simulink model "BLDCmotorControl_FOC_R2017b_fixdt_Ffwd"  (R2025a)
settings: Solver=FixedStepDiscrete  StartTime=0  StopTime=0.5  FixedStep=Ts  MaxStep=1e-6  RelTol=1e-6  AbsTol=1e-6  EnableMultiTasking=on
PreLoadFcn:
  | addpath(genpath('01_Libraries'));
  | addpath(genpath('02_Figures'));
InitFcn:
  | init_model;
undefined symbols (not defined in the file): a_elecAngle, b_DCLinkCurrAvail, b_diagEna, b_FfwdEna, b_fieldWeakEna, b_selPhaABCurrMeas, cf_currFilt, cf_speedCoef, cf_speedFilt, CTRL_COM, DiscIntNeverNeededParam, dV_openRate, DWORK0, DWORK1, DWORK2, DWORK3, dz_cntTrnsDetHi, dz_cntTrnsDetLo, i_errThres, i_max, i_thresOutlier, id_fieldWeak_M1, id_Kb, id_Ki, id_Kp, iq_Kb, iq_Ki, iq_KiLimProt, iq_Kp, iq_KpLimProt, iq_max_M1, Ld, Lq, mot_lambda, mot_Ld, mot_Lq, n_commAcvLo, n_commDeacvHi, n_Kb, n_Ki, n_Kp, n_KpLimProt, n_max, n_stdStillDet, OPEN_MODE, r_cos_M1, r_sin_M1, r_whl, Rs, SPD_MODE, t_errDequal, t_errQual, TRQ_MODE, Ts, Ts_ctrl, V_max, V_min, Vd_max, vec_hallToPos, VLT_MODE ... (+5)
libraries: BLDC_controller_Lib x12, simulink x11, spsPermanentMagnetSynchronousMachineLib x4, spsVoltageMeasurementLib x4, spsControlledVoltageSourceLib x2, spsUniversalBridgeLib x2, spspowerguiLib x2, eePwmGenerator x1, SignalEditorBlockLib x1
(part 2 of 4)

== system BLDCmotorControl_FOC_R2017b_fixdt_Ffwd/PWM_gates/PWM_generator12 ==
  DC : Inport  SampleTime=Ts
  PWM_generator_sfcn : S-Function  FunctionName=PWM_generator_sf  SFunctionModules=""  SFunctionDeploymentMode=off  EnableBusSupport=off  SFcnStateName=DWORK0  mask{rtw_sf_name=PWM_generator_sf, showVar=off}
      mask prompts: rtw_sf_name "Simulink:masks:GenSFuncName_MP"; showVar "Simulink:masks:GenSFuncShowModuleList_MP"
      mask help: Simulink:masks:GenSFuncDesc_MD
      mask init: same as BLDCmotorControl_FOC_R2017b_fixdt_Ffwd/BLDC_model_closed/BLDC_model_sfcn
      settings: SFcnIsStateOwnerBlock=on
      settings: CopyFcn=|
      | if ~strcmp(get_param(gcb,'Linkstatus'),'none') && ...
      | ~strcmp(get_param(gcb,'Linkstatus'),'implicit')
      |   set_param(gcb,'LinkStatus','none');
      | end
      mask Help: eval('feval(''rtwprivate'',''rtwhelpview'',''rtw_sfcn_block'')');
      mask Display:
      | port_label('input',1,'DC');
      | port_label('output',1,'PWM');
  __InputSSForSFun__ : Subsystem
  __OutputSSForSFun__ : Subsystem
  PWM : Outport  VectorParamsAs1DForOutWhenUnconnected=off
  wires:
  DC/1 -> __InputSSForSFun__/1(DC)
  __InputSSForSFun__/1(__UniqueOutportName__1__) -> PWM_generator_sfcn/1
  PWM_generator_sfcn/1 -> __OutputSSForSFun__/1(__UniqueInportName__1__)
  __OutputSSForSFun__/1(PWM) -> PWM/1

== system BLDCmotorControl_FOC_R2017b_fixdt_Ffwd/PWM_gates/PWM_generator2 ==
  DC : Inport  SampleTime=Ts
  PWM_generator_sfcn : S-Function  FunctionName=PWM_generator_sf  SFunctionModules=""  SFunctionDeploymentMode=off  EnableBusSupport=off  SFcnStateName=DWORK0  mask{rtw_sf_name=PWM_generator_sf, showVar=off}
      mask prompts: rtw_sf_name "Simulink:masks:GenSFuncName_MP"; showVar "Simulink:masks:GenSFuncShowModuleList_MP"
      mask help: Simulink:masks:GenSFuncDesc_MD
      mask init: same as BLDCmotorControl_FOC_R2017b_fixdt_Ffwd/BLDC_model_closed/BLDC_model_sfcn
      settings: SFcnIsStateOwnerBlock=on
      settings: CopyFcn=|
      | if ~strcmp(get_param(gcb,'Linkstatus'),'none') && ...
      | ~strcmp(get_param(gcb,'Linkstatus'),'implicit')
      |   set_param(gcb,'LinkStatus','none');
      | end
      mask Help: eval('feval(''rtwprivate'',''rtwhelpview'',''rtw_sfcn_block'')');
      mask Display:
      | port_label('input',1,'DC');
      | port_label('output',1,'PWM');
  __InputSSForSFun__ : Subsystem
  __OutputSSForSFun__ : Subsystem
  PWM : Outport  VectorParamsAs1DForOutWhenUnconnected=off
  wires:
  DC/1 -> __InputSSForSFun__/1(DC)
  __InputSSForSFun__/1(__UniqueOutportName__1__) -> PWM_generator_sfcn/1
  PWM_generator_sfcn/1 -> __OutputSSForSFun__/1(__UniqueInportName__1__)
  __OutputSSForSFun__/1(PWM) -> PWM/1

== system BLDCmotorControl_FOC_R2017b_fixdt_Ffwd/PWM_gates/PWM_generator3 ==
  DC : Inport  SampleTime=Ts
  PWM_generator_sfcn : S-Function  FunctionName=PWM_generator_sf  SFunctionModules=""  SFunctionDeploymentMode=off  EnableBusSupport=off  SFcnStateName=DWORK0  mask{rtw_sf_name=PWM_generator_sf, showVar=off}
      mask prompts: rtw_sf_name "Simulink:masks:GenSFuncName_MP"; showVar "Simulink:masks:GenSFuncShowModuleList_MP"
      mask help: Simulink:masks:GenSFuncDesc_MD
      mask init: same as BLDCmotorControl_FOC_R2017b_fixdt_Ffwd/BLDC_model_closed/BLDC_model_sfcn
      settings: SFcnIsStateOwnerBlock=on
      settings: CopyFcn=|
      | if ~strcmp(get_param(gcb,'Linkstatus'),'none') && ...
      | ~strcmp(get_param(gcb,'Linkstatus'),'implicit')
      |   set_param(gcb,'LinkStatus','none');
      | end
      mask Help: eval('feval(''rtwprivate'',''rtwhelpview'',''rtw_sfcn_block'')');
      mask Display:
      | port_label('input',1,'DC');
      | port_label('output',1,'PWM');
  __InputSSForSFun__ : Subsystem
  __OutputSSForSFun__ : Subsystem
  PWM : Outport  VectorParamsAs1DForOutWhenUnconnected=off
  wires:
  __OutputSSForSFun__/1(PWM) -> PWM/1
  PWM_generator_sfcn/1 -> __OutputSSForSFun__/1(__UniqueInportName__1__)
  __InputSSForSFun__/1(__UniqueOutportName__1__) -> PWM_generator_sfcn/1
  DC/1 -> __InputSSForSFun__/1(DC)

== system BLDCmotorControl_FOC_R2017b_fixdt_Ffwd/PWM_gates/PWM_generator4 ==
  DC : Inport  SampleTime=Ts
  PWM_generator_sfcn : S-Function  FunctionName=PWM_generator_sf  SFunctionModules=""  SFunctionDeploymentMode=off  EnableBusSupport=off  SFcnStateName=DWORK0  mask{rtw_sf_name=PWM_generator_sf, showVar=off}
      mask prompts: rtw_sf_name "Simulink:masks:GenSFuncName_MP"; showVar "Simulink:masks:GenSFuncShowModuleList_MP"
      mask help: Simulink:masks:GenSFuncDesc_MD
      mask init: same as BLDCmotorControl_FOC_R2017b_fixdt_Ffwd/BLDC_model_closed/BLDC_model_sfcn
      settings: SFcnIsStateOwnerBlock=on
      settings: CopyFcn=|
      | if ~strcmp(get_param(gcb,'Linkstatus'),'none') && ...
      | ~strcmp(get_param(gcb,'Linkstatus'),'implicit')
      |   set_param(gcb,'LinkStatus','none');
      | end
      mask Help: eval('feval(''rtwprivate'',''rtwhelpview'',''rtw_sfcn_block'')');
      mask Display:
      | port_label('input',1,'DC');
      | port_label('output',1,'PWM');
  __InputSSForSFun__ : Subsystem
  __OutputSSForSFun__ : Subsystem
  PWM : Outport  VectorParamsAs1DForOutWhenUnconnected=off
  wires:
  DC/1 -> __InputSSForSFun__/1(DC)
  __InputSSForSFun__/1(__UniqueOutportName__1__) -> PWM_generator_sfcn/1
  PWM_generator_sfcn/1 -> __OutputSSForSFun__/1(__UniqueInportName__1__)
  __OutputSSForSFun__/1(PWM) -> PWM/1

== system BLDCmotorControl_FOC_R2017b_fixdt_Ffwd/PWM_gates/PWM_generator5 ==
  DC : Inport  SampleTime=Ts
  PWM_generator_sfcn : S-Function  FunctionName=PWM_generator_sf  SFunctionModules=""  SFunctionDeploymentMode=off  EnableBusSupport=off  SFcnStateName=DWORK0  mask{rtw_sf_name=PWM_generator_sf, showVar=off}
      mask prompts: rtw_sf_name "Simulink:masks:GenSFuncName_MP"; showVar "Simulink:masks:GenSFuncShowModuleList_MP"
      mask help: Simulink:masks:GenSFuncDesc_MD
      mask init: same as BLDCmotorControl_FOC_R2017b_fixdt_Ffwd/BLDC_model_closed/BLDC_model_sfcn
      settings: SFcnIsStateOwnerBlock=on
      settings: CopyFcn=|
      | if ~strcmp(get_param(gcb,'Linkstatus'),'none') && ...
      | ~strcmp(get_param(gcb,'Linkstatus'),'implicit')
      |   set_param(gcb,'LinkStatus','none');
      | end
      mask Help: eval('feval(''rtwprivate'',''rtwhelpview'',''rtw_sfcn_block'')');
      mask Display:
      | port_label('input',1,'DC');
      | port_label('output',1,'PWM');
  __InputSSForSFun__ : Subsystem
  __OutputSSForSFun__ : Subsystem
  PWM : Outport  VectorParamsAs1DForOutWhenUnconnected=off
  wires:
  __OutputSSForSFun__/1(PWM) -> PWM/1
  PWM_generator_sfcn/1 -> __OutputSSForSFun__/1(__UniqueInportName__1__)
  __InputSSForSFun__/1(__UniqueOutportName__1__) -> PWM_generator_sfcn/1
  DC/1 -> __InputSSForSFun__/1(DC)

== system BLDCmotorControl_FOC_R2017b_fixdt_Ffwd/PWM_gates/signal_log6 ==
  PWM : Inport
  Terminator_1 : Terminator
  wires:
  PWM/1 -> Terminator_1/1  "PWM"

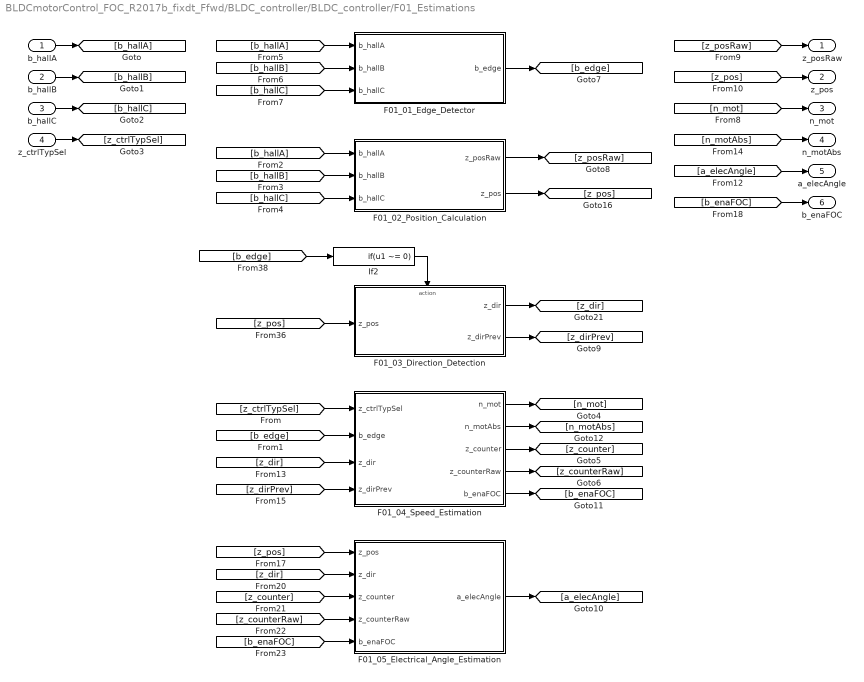
== system BLDCmotorControl_FOC_R2017b_fixdt_Ffwd/BLDC_controller/BLDC_controller/F01_Estimations ==
  b_hallA : Inport
  b_hallB : Inport  Port=2
  b_hallC : Inport  Port=3
  z_ctrlTypSel : Inport  Port=4
  F01_01_Edge_Detector : Subsystem
  F01_02_Position_Calculation : Subsystem
  F01_03_Direction_Detection : Subsystem
  F01_04_Speed_Estimation : Subsystem
  F01_05_Electrical_Angle_Estimation : Subsystem
  If2 : If  IfExpression=u1 ~= 0  ShowElse=off
  z_posRaw : Outport  OutputWhenDisabled=reset  InitialOutput=0  VectorParamsAs1DForOutWhenUnconnected=off
  z_pos : Outport  Port=2  OutputWhenDisabled=reset  InitialOutput=0  VectorParamsAs1DForOutWhenUnconnected=off
  "n_mot " : Outport  Port=3  OutputWhenDisabled=reset  InitialOutput=0  VectorParamsAs1DForOutWhenUnconnected=off
  n_motAbs : Outport  Port=4  OutputWhenDisabled=reset  InitialOutput=0  VectorParamsAs1DForOutWhenUnconnected=off
  a_elecAngle : Outport  Port=5  OutputWhenDisabled=reset  InitialOutput=0  VectorParamsAs1DForOutWhenUnconnected=off
  b_enaFOC : Outport  Port=6  VectorParamsAs1DForOutWhenUnconnected=off
  wires:
  If2/1 -> F01_03_Direction_Detection/Action
  [b_edge] -> If2/1
  [z_pos] -> F01_03_Direction_Detection/1(z_pos)
  [b_hallA] -> F01_01_Edge_Detector/1(b_hallA)
  F01_01_Edge_Detector/1("b_edge ") -> [b_edge]
  F01_03_Direction_Detection/1(z_dir) -> [z_dir]
  [b_hallB] -> F01_01_Edge_Detector/2(b_hallB)
  [b_hallC] -> F01_01_Edge_Detector/3(b_hallC)
  b_hallA/1 -> [b_hallA]
  b_hallB/1 -> [b_hallB]
  b_hallC/1 -> [b_hallC]
  [b_hallC] -> F01_02_Position_Calculation/3(b_hallC)
  [b_hallB] -> F01_02_Position_Calculation/2(b_hallB)
  [b_hallA] -> F01_02_Position_Calculation/1(b_hallA)
  F01_02_Position_Calculation/2("z_pos ") -> [z_pos]
  [b_edge] -> F01_04_Speed_Estimation/2(b_edge)
  F01_04_Speed_Estimation/1(n_mot) -> [n_mot]
  [n_mot] -> "n_mot "/1
  [z_pos] -> z_pos/1
  [z_dir] -> F01_04_Speed_Estimation/3(z_dir)
  F01_04_Speed_Estimation/3(z_counter) -> [z_counter]
  F01_04_Speed_Estimation/4(z_counterRaw) -> [z_counterRaw]
  F01_03_Direction_Detection/2(z_dirPrev) -> [z_dirPrev]
  [z_dirPrev] -> F01_04_Speed_Estimation/4(z_dirPrev)
  [z_pos] -> F01_05_Electrical_Angle_Estimation/1(z_pos)
  [z_dir] -> F01_05_Electrical_Angle_Estimation/2(z_dir)
  [z_counter] -> F01_05_Electrical_Angle_Estimation/3(z_counter)
  [z_counterRaw] -> F01_05_Electrical_Angle_Estimation/4(z_counterRaw)
  [b_enaFOC] -> F01_05_Electrical_Angle_Estimation/5(b_enaFOC)
  F01_04_Speed_Estimation/5(b_enaFOC) -> [b_enaFOC]
  [z_ctrlTypSel] -> F01_04_Speed_Estimation/1(z_ctrlTypSel)
  [b_enaFOC] -> b_enaFOC/1
  [a_elecAngle] -> a_elecAngle/1
  F01_05_Electrical_Angle_Estimation/1(a_elecAngle) -> [a_elecAngle]
  F01_04_Speed_Estimation/2(n_motAbs) -> [n_motAbs]
  [n_motAbs] -> n_motAbs/1
  z_ctrlTypSel/1 -> [z_ctrlTypSel]
  F01_02_Position_Calculation/1(z_posRaw) -> [z_posRaw]
  [z_posRaw] -> z_posRaw/1

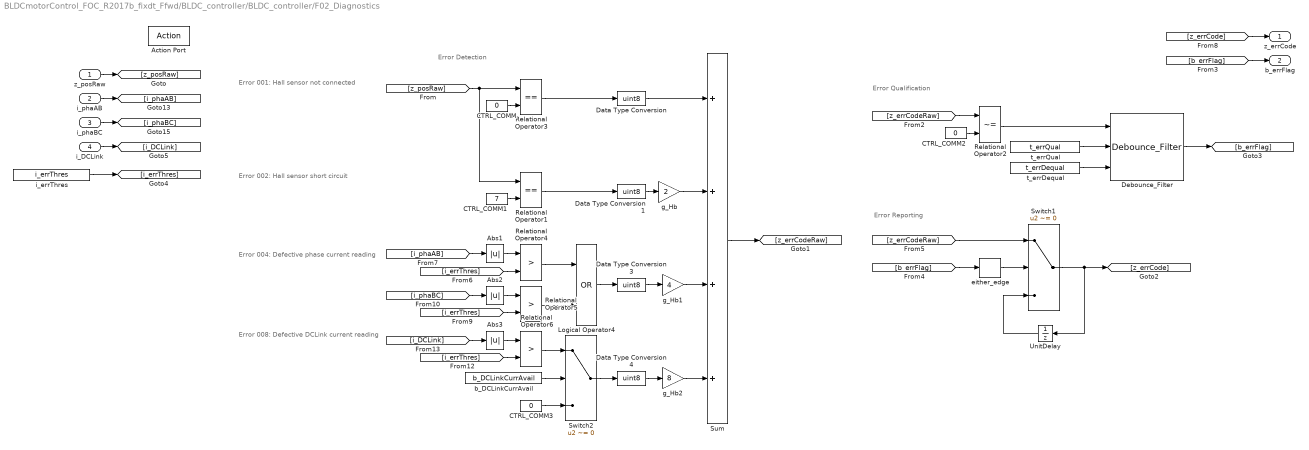
== system BLDCmotorControl_FOC_R2017b_fixdt_Ffwd/BLDC_controller/BLDC_controller/F02_Diagnostics ==
  note: Error 001: Hall sensor not connected
  note: Error 002: Hall sensor short circuit
  note: Error Qualification
  note: Error Detection
  note: Error Reporting
  note: Error 004: Defective phase current reading
  note: Error 008: Defective DCLink current reading
  z_posRaw : Inport
  i_phaAB : Inport  Port=2
  i_phaBC : Inport  Port=3
  i_DCLink : Inport  Port=4
  Action Port : ActionPort  InitializeStates=reset  ActionPortLabel=if { }
  Abs1 : Abs  SaturateOnIntegerOverflow=off
  Abs2 : Abs  SaturateOnIntegerOverflow=off
  Abs3 : Abs  SaturateOnIntegerOverflow=off
  CTRL_COMM : Constant  Value=0  OutDataTypeStr=Inherit: Inherit via back propagation
  CTRL_COMM1 : Constant  Value=7  OutDataTypeStr=Inherit: Inherit via back propagation
  CTRL_COMM2 : Constant  Value=0  OutDataTypeStr=Inherit: Inherit via back propagation
  CTRL_COMM3 : Constant  Value=0  OutDataTypeStr=Inherit: Inherit via back propagation
  Data Type Conversion{,1,3..4} (4 alike) : DataTypeConversion  OutDataTypeStr=uint8  SaturateOnIntegerOverflow=off  RndMeth=Floor
  Debounce_Filter : BLDC_controller_Lib/Debounce_Filter
  Logical Operator4 : Logic  Operator=OR  AllPortsSameDT=off  OutDataTypeStr=boolean
  Relational Operator1 : RelationalOperator  Operator===  OutDataTypeStr=boolean  RndMeth=Simplest  InputSameDT=off
  Relational Operator2 : RelationalOperator  Operator=~=  OutDataTypeStr=boolean  RndMeth=Simplest  InputSameDT=off
  Relational Operator3 : RelationalOperator  Operator===  OutDataTypeStr=boolean  RndMeth=Simplest  InputSameDT=off
  Relational Operator4 : RelationalOperator  Operator=>  OutDataTypeStr=boolean  RndMeth=Simplest  InputSameDT=off
  Relational Operator5 : RelationalOperator  Operator=>  OutDataTypeStr=boolean  RndMeth=Simplest  InputSameDT=off
  Relational Operator6 : RelationalOperator  Operator=>  OutDataTypeStr=boolean  RndMeth=Simplest  InputSameDT=off
  Sum : Sum  Inputs=++++  RndMeth=Simplest  OutDataTypeStr=Inherit: Same as first input
  Switch1 : Switch  Criteria=u2 ~= 0  OutDataTypeStr=Inherit: Inherit via back propagation  RndMeth=Zero  SaturateOnIntegerOverflow=off  InputSameDT=off
  Switch2 : Switch  Criteria=u2 ~= 0  OutDataTypeStr=Inherit: Inherit via back propagation  RndMeth=Zero  SaturateOnIntegerOverflow=off  InputSameDT=off
  UnitDelay : UnitDelay  SampleTime=-1  HasFrameUpgradeWarning=on
      settings: AttributesFormatString=Ini=%<X0>
  b_DCLinkCurrAvail : Constant  Value=b_DCLinkCurrAvail  OutDataTypeStr=boolean
  either_edge : BLDC_controller_Lib/either_edge
  g_Hb : Gain  Gain=2  RndMeth=Simplest  OutDataTypeStr=Inherit: Same as input
  g_Hb1 : Gain  Gain=4  RndMeth=Simplest  OutDataTypeStr=Inherit: Same as input
  g_Hb2 : Gain  Gain=8  RndMeth=Simplest  OutDataTypeStr=Inherit: Same as input
  i_errThres : Constant  Value=i_errThres  OutDataTypeStr=Inherit: Inherit via back propagation
  t_errDequal : Constant  Value=t_errDequal  OutDataTypeStr=Inherit: Inherit via back propagation
  t_errQual : Constant  Value=t_errQual  OutDataTypeStr=Inherit: Inherit via back propagation
  "z_errCode " : Outport  OutputWhenDisabled=reset  InitialOutput=0  VectorParamsAs1DForOutWhenUnconnected=off
  b_errFlag : Outport  Port=2  OutputWhenDisabled=reset  InitialOutput=0  VectorParamsAs1DForOutWhenUnconnected=off
  wires:
  [z_errCode] -> "z_errCode "/1
  z_posRaw/1 -> [z_posRaw]
  t_errDequal/1 -> Debounce_Filter/3
  t_errQual/1 -> Debounce_Filter/2
  CTRL_COMM/1 -> Relational Operator3/2
  CTRL_COMM1/1 -> Relational Operator1/2
  [z_posRaw] -> Relational Operator1/1, Relational Operator3/1
  Relational Operator3/1 -> Data Type Conversion/1
  Sum/1 -> [z_errCodeRaw]
  Relational Operator2/1 -> Debounce_Filter/1
  [z_errCodeRaw] -> Relational Operator2/1
  CTRL_COMM2/1 -> Relational Operator2/2
  Debounce_Filter/1 -> [b_errFlag]
  either_edge/1 -> Switch1/2
  UnitDelay/1 -> Switch1/3
  Switch1/1 -> UnitDelay/1, [z_errCode]
  [b_errFlag] -> b_errFlag/1
  [b_errFlag] -> either_edge/1
  [z_errCodeRaw] -> Switch1/1
  i_DCLink/1 -> [i_DCLink]
  i_phaBC/1 -> [i_phaBC]
  i_phaAB/1 -> [i_phaAB]
  [i_errThres] -> Relational Operator4/2
  Abs1/1 -> Relational Operator4/1
  g_Hb/1 -> Sum/2
  Relational Operator1/1 -> Data Type Conversion1/1
  Data Type Conversion/1 -> Sum/1
  Data Type Conversion1/1 -> g_Hb/1
  [i_phaAB] -> Abs1/1
  i_errThres/1 -> [i_errThres]
  Relational Operator4/1 -> Logical Operator4/1
  [i_phaBC] -> Abs2/1
  Abs2/1 -> Relational Operator5/1
  [i_errThres] -> Relational Operator5/2
  Relational Operator5/1 -> Logical Operator4/2
  Logical Operator4/1 -> Data Type Conversion3/1
  Data Type Conversion3/1 -> g_Hb1/1
  g_Hb1/1 -> Sum/3
  [i_errThres] -> Relational Operator6/2
  Abs3/1 -> Relational Operator6/1
  [i_DCLink] -> Abs3/1
  b_DCLinkCurrAvail/1 -> Switch2/2
  g_Hb2/1 -> Sum/4
  Data Type Conversion4/1 -> g_Hb2/1
  Relational Operator6/1 -> Switch2/1
  CTRL_COMM3/1 -> Switch2/3
  Switch2/1 -> Data Type Conversion4/1

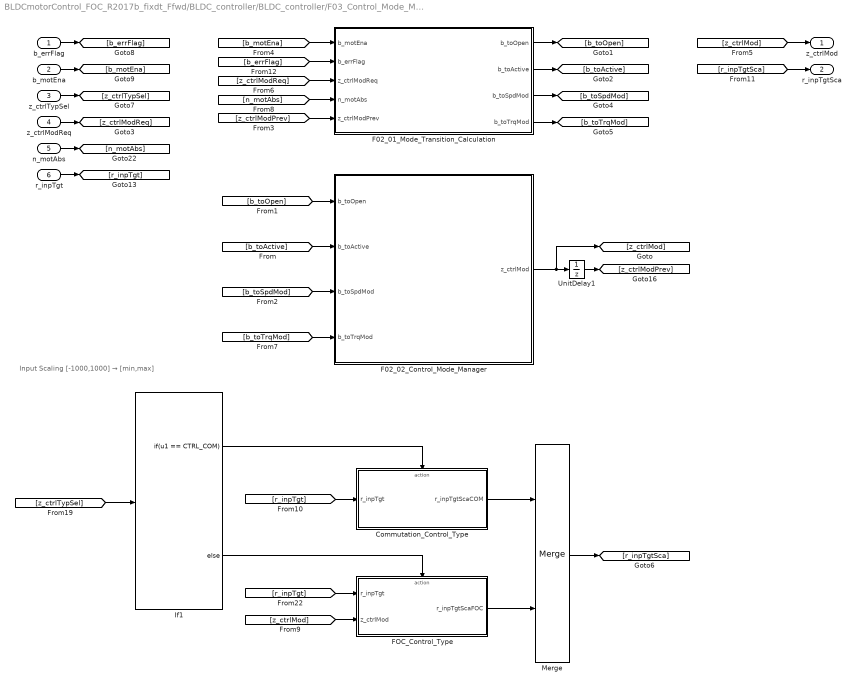
== system BLDCmotorControl_FOC_R2017b_fixdt_Ffwd/BLDC_controller/BLDC_controller/F03_Control_Mode_Manager ==
  note: Input Scaling [-1000,1000] → [min,max]
  b_errFlag : Inport
  b_motEna : Inport  Port=2
  z_ctrlTypSel : Inport  Port=3
  z_ctrlModReq : Inport  Port=4
  n_motAbs : Inport  Port=5
  r_inpTgt : Inport  Port=6
  Commutation_Control_Type : Subsystem
  F02_01_Mode_Transition_Calculation : Subsystem
  F02_02_Control_Mode_Manager : Stateflow chart  TreatAsAtomicUnit=on
  FOC_Control_Type : Subsystem
  If1 : If  IfExpression=u1 == CTRL_COM
  Merge : Merge
  UnitDelay1 : UnitDelay  SampleTime=-1  HasFrameUpgradeWarning=on
  z_ctrlMod : Outport  OutputWhenDisabled=reset  InitialOutput=0  VectorParamsAs1DForOutWhenUnconnected=off
  r_inpTgtSca : Outport  Port=2  OutputWhenDisabled=reset  InitialOutput=0  VectorParamsAs1DForOutWhenUnconnected=off
  wires:
  [z_ctrlMod] -> z_ctrlMod/1
  b_motEna/1 -> [b_motEna]
  [b_toOpen] -> F02_02_Control_Mode_Manager/1(b_toOpen)
  [b_toSpdMod] -> F02_02_Control_Mode_Manager/3(b_toSpdMod)
  z_ctrlModReq/1 -> [z_ctrlModReq]
  [b_toTrqMod] -> F02_02_Control_Mode_Manager/4(b_toTrqMod)
  UnitDelay1/1 -> [z_ctrlModPrev]
  F02_02_Control_Mode_Manager/1(z_ctrlMod) -> [z_ctrlMod], UnitDelay1/1
  n_motAbs/1 -> [n_motAbs]
  [b_toActive] -> F02_02_Control_Mode_Manager/2(b_toActive)
  F02_01_Mode_Transition_Calculation/1(b_toOpen) -> [b_toOpen]
  F02_01_Mode_Transition_Calculation/2(b_toActive) -> [b_toActive]
  F02_01_Mode_Transition_Calculation/3(b_toSpdMod) -> [b_toSpdMod]
  F02_01_Mode_Transition_Calculation/4(b_toTrqMod) -> [b_toTrqMod]
  [z_ctrlModPrev] -> F02_01_Mode_Transition_Calculation/5(z_ctrlModPrev)
  [b_motEna] -> F02_01_Mode_Transition_Calculation/1(b_motEna)
  [z_ctrlModReq] -> F02_01_Mode_Transition_Calculation/3(z_ctrlModReq)
  [n_motAbs] -> F02_01_Mode_Transition_Calculation/4(n_motAbs)
  [z_ctrlTypSel] -> If1/1
  [z_ctrlMod] -> FOC_Control_Type/2(z_ctrlMod)
  [r_inpTgt] -> FOC_Control_Type/1(r_inpTgt)
  If1/1 -> Commutation_Control_Type/Action
  [r_inpTgt] -> Commutation_Control_Type/1(r_inpTgt)
  If1/2 -> FOC_Control_Type/Action
  Commutation_Control_Type/1(r_inpTgtScaCOM) -> Merge/1
  FOC_Control_Type/1(r_inpTgtScaFOC) -> Merge/2
  Merge/1 -> [r_inpTgtSca]
  [r_inpTgtSca] -> r_inpTgtSca/1
  z_ctrlTypSel/1 -> [z_ctrlTypSel]
  r_inpTgt/1 -> [r_inpTgt]
  b_errFlag/1 -> [b_errFlag]
  [b_errFlag] -> F02_01_Mode_Transition_Calculation/2(b_errFlag)

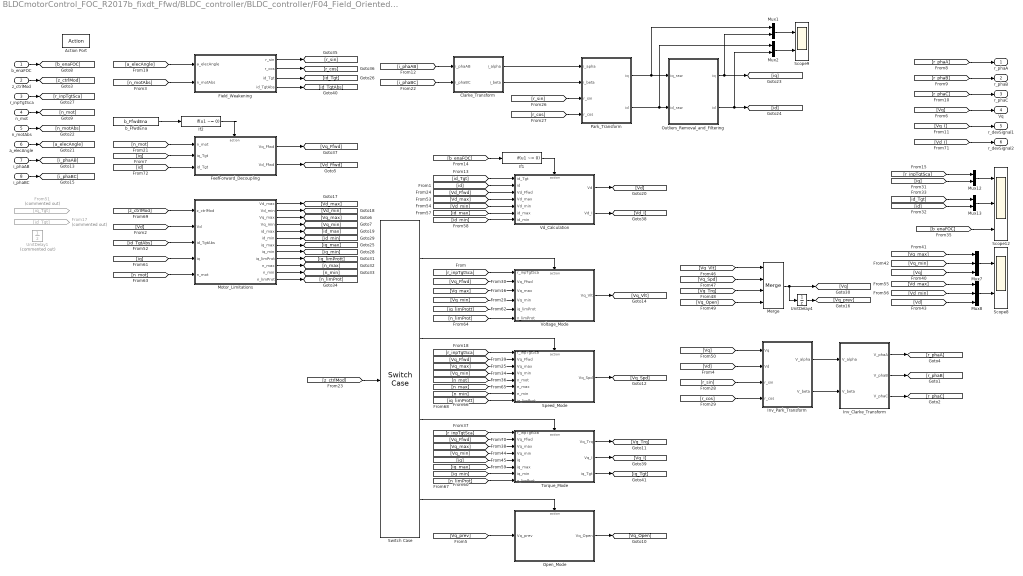
== system BLDCmotorControl_FOC_R2017b_fixdt_Ffwd/BLDC_controller/BLDC_controller/F04_Field_Oriented_Control ==
  b_enaFOC : Inport
  z_ctrlMod : Inport  Port=2
  r_inpTgtSca : Inport  Port=3
  n_mot : Inport  Port=4
  n_motAbs : Inport  Port=5
  a_elecAngle : Inport  Port=6
  i_phaAB : Inport  Port=7
  i_phaBC : Inport  Port=8
  Action Port : ActionPort  InitializeStates=reset  ActionPortLabel=if { }
  Clarke_Transform : Subsystem
  FeefForward_Decoupling : Subsystem
  Field_Weakening : Subsystem
  From17 : From  Commented=on  GotoTag=id_Tgt
  From51 : From  Commented=on  GotoTag=iq_Tgt
  If1 : If  IfExpression=u1 ~= 0  ShowElse=off
  If2 : If  IfExpression=u1 ~= 0  ShowElse=off
  Inv_Clarke_Transform : Subsystem
  Inv_Park_Transform : Subsystem
  Merge : Merge  Inputs=4
  Motor_Limitations : Subsystem
  Mux{1..2,12..13} (4 alike) : Mux  Inputs=2
  Mux7 : Mux  Inputs=3
  Mux8 : Mux  Inputs=3
  Open_Mode : Subsystem
  Outliers_Removal_and_Filtering : Subsystem
  Park_Transform : Subsystem
  Scope12 : Scope  NumInputPorts=3
      settings: ActiveDisplayYMinimum=-1321.53125  ActiveDisplayYMaximum=1255.65625  DataLoggingVariableName=ScopeData11
  Scope8 : Scope  NumInputPorts=2
      settings: ActiveDisplayYMinimum=-1125  ActiveDisplayYMaximum=1125
  Scope9 : Scope  NumInputPorts=2
      settings: ActiveDisplayYMinimum=-2209.89844  ActiveDisplayYMaximum=1912.21094  DataLoggingVariableName=ScopeData3
  Speed_Mode : Subsystem
  Switch Case : SwitchCase  CaseConditions={VLT_MODE, SPD_MODE, TRQ_MODE}
  Torque_Mode : Subsystem
  UnitDelay1 : UnitDelay  Commented=on  SampleTime=-1  HasFrameUpgradeWarning=on
      settings: AttributesFormatString=Ini=%<X0>
  UnitDelay4 : UnitDelay  SampleTime=-1  HasFrameUpgradeWarning=on
      settings: AttributesFormatString=Ini=%<X0>
  Vd_Calculation : Subsystem
  Voltage_Mode : Subsystem
  b_FfwdEna : Constant  Value=b_FfwdEna  OutDataTypeStr=boolean
  r_phaA : Outport  OutputWhenDisabled=reset  InitialOutput=0  VectorParamsAs1DForOutWhenUnconnected=off
  r_phaB : Outport  Port=2  OutputWhenDisabled=reset  InitialOutput=0  VectorParamsAs1DForOutWhenUnconnected=off
  "r_phaC " : Outport  Port=3  OutputWhenDisabled=reset  InitialOutput=0  VectorParamsAs1DForOutWhenUnconnected=off
  Vq : Outport  Port=4  OutputWhenDisabled=reset  InitialOutput=0  VectorParamsAs1DForOutWhenUnconnected=off
  r_devSignal1 : Outport  Port=5  OutputWhenDisabled=reset  InitialOutput=0  VectorParamsAs1DForOutWhenUnconnected=off
  r_devSignal2 : Outport  Port=6  OutputWhenDisabled=reset  InitialOutput=0  VectorParamsAs1DForOutWhenUnconnected=off
  wires:
  [r_phaA] -> r_phaA/1
  [r_phaB] -> r_phaB/1
  [r_phaC] -> "r_phaC "/1
  Inv_Park_Transform/1(V_alpha) -> Inv_Clarke_Transform/1(V_alpha)
  Inv_Park_Transform/2(V_beta) -> Inv_Clarke_Transform/2(V_beta)
  i_phaAB/1 -> [i_phaAB]
  i_phaBC/1 -> [i_phaBC]
  Inv_Clarke_Transform/1(V_phaA) -> [r_phaA]
  Inv_Clarke_Transform/2(V_phaB) -> [r_phaB]
  Inv_Clarke_Transform/3(V_phaC) -> [r_phaC]
  Clarke_Transform/1(i_alpha) -> Park_Transform/1(i_apha)
  Clarke_Transform/2(i_beta) -> Park_Transform/2(i_beta)
  Mux12/1 -> Scope12/1
  Mux13/1 -> Scope12/2
  [r_sin] -> Park_Transform/3(r_sin)
  [r_cos] -> Park_Transform/4(r_cos)
  [r_sin] -> Inv_Park_Transform/3(r_sin)
  [r_cos] -> Inv_Park_Transform/4(r_cos)
  [r_inpTgtSca] -> Mux12/1
  [iq] -> Mux12/2
  [id] -> Mux13/2
  [id_Tgt] -> Mux13/1
  r_inpTgtSca/1 -> [r_inpTgtSca]
  [i_phaAB] -> Clarke_Transform/1(i_phaAB)
  [i_phaBC] -> Clarke_Transform/2(i_phaBC)
  [Vd_max] -> Mux8/1
  [Vd] -> Mux8/3
  Mux8/1 -> Scope8/2
  [Vd_min] -> Mux8/2
  [Vq] -> Mux7/3
  Mux7/1 -> Scope8/1
  [Vq_max] -> Mux7/1
  [Vq_min] -> Mux7/2
  Park_Transform/2(id) -> Outliers_Removal_and_Filtering/2(id_raw), Mux2/1
  Park_Transform/1(iq) -> Outliers_Removal_and_Filtering/1(iq_raw), Mux1/1
  Outliers_Removal_and_Filtering/1(iq) -> [iq], Mux1/2
  Outliers_Removal_and_Filtering/2(id) -> [id], Mux2/2
  [Vq] -> Vq/1
  Vd_Calculation/1(Vd) -> [Vd]
  [id] -> Vd_Calculation/2(id)
  [id_Tgt] -> Vd_Calculation/1(id_Tgt)
  b_enaFOC/1 -> [b_enaFOC]
  If1/1 -> Vd_Calculation/Action
  [b_enaFOC] -> If1/1
  [Vd] -> Inv_Park_Transform/2(Vd)
  z_ctrlMod/1 -> [z_ctrlMod]
  n_mot/1 -> [n_mot]
  [b_enaFOC] -> Scope12/3
  [z_ctrlMod] -> Switch Case/1
  [Vq_prev] -> Open_Mode/1(Vq_prev)
  Open_Mode/1(Vq_Open) -> [Vq_Open]
  Torque_Mode/1(Vq_Trq) -> [Vq_Trq]
  Speed_Mode/1(Vq_Spd) -> [Vq_Spd]
  Voltage_Mode/1(Vq_Vlt) -> [Vq_Vlt]
  [r_inpTgtSca] -> Voltage_Mode/1(r_inpTgtSca)
  [Vq_max] -> Voltage_Mode/3(Vq_max)
  [Vq_min] -> Voltage_Mode/4(Vq_min)
  [r_inpTgtSca] -> Speed_Mode/1(r_inpTgtSca)
  [Vq_max] -> Speed_Mode/3(Vq_max)
  [Vq_min] -> Speed_Mode/4(Vq_min)
  [n_mot] -> Speed_Mode/5(n_mot)
  [Vq_min] -> Torque_Mode/4(Vq_min)
  [Vq_max] -> Torque_Mode/3(Vq_max)
  [r_inpTgtSca] -> Torque_Mode/1(r_inpTgtSca)
  [iq] -> Torque_Mode/5(iq)
  Switch Case/1 -> Voltage_Mode/Action
  Switch Case/2 -> Speed_Mode/Action
  Switch Case/3 -> Torque_Mode/Action
  Switch Case/4 -> Open_Mode/Action
  [Vq_Vlt] -> Merge/1
  [Vq_Spd] -> Merge/2
  [Vq_Trq] -> Merge/3
  [Vq_Open] -> Merge/4
  [Vq] -> Inv_Park_Transform/1(Vq)
  Merge/1 -> UnitDelay4/1, [Vq]
  UnitDelay4/1 -> [Vq_prev]
  Motor_Limitations/3(Vq_max) -> [Vq_max]
  Motor_Limitations/4(Vq_min) -> [Vq_min]
  [Vd] -> Motor_Limitations/2(Vd)
  [id_TgtAbs] -> Motor_Limitations/3(id_TgtAbs)
  Motor_Limitations/2(Vd_min) -> [Vd_min]
  Motor_Limitations/1(Vd_max) -> [Vd_max]
  [Vd_max] -> Vd_Calculation/4(Vd_max)
  [Vd_min] -> Vd_Calculation/5(Vd_min)
  Motor_Limitations/5(id_max) -> [id_max]
  Motor_Limitations/6(id_min) -> [id_min]
  Motor_Limitations/7(iq_max) -> [iq_max]
  Motor_Limitations/8(iq_min) -> [iq_min]
  [id_max] -> Vd_Calculation/6(id_max)
  [id_min] -> Vd_Calculation/7(id_min)
  [iq_max] -> Torque_Mode/6(iq_max)
  [iq_min] -> Torque_Mode/7(iq_min)
  [iq] -> Motor_Limitations/4(iq)
  Motor_Limitations/9(iq_limProt) -> [iq_limPrott]
  [iq_limPrott] -> Voltage_Mode/5(iq_limProt)
  Motor_Limitations/11(n_min) -> [n_min]
  Motor_Limitations/10(n_max) -> [n_max]
  Motor_Limitations/12(n_limProt) -> [n_limProt]
  [n_mot] -> Motor_Limitations/5(n_mot)
  [n_limProt] -> Voltage_Mode/6(n_limProt)
  [n_max] -> Speed_Mode/6(n_max)
  [n_min] -> Speed_Mode/7(n_min)
  [n_limProt] -> Torque_Mode/8(n_limProt)
  [iq_limPrott] -> Speed_Mode/8(iq_limProt)
  [z_ctrlMod] -> Motor_Limitations/1(z_ctrlMod)
  n_motAbs/1 -> [n_motAbs]
  Field_Weakening/1(r_sin) -> [r_sin]
  Field_Weakening/2(r_cos) -> [r_cos]
  [a_elecAngle] -> Field_Weakening/1(a_elecAngle)
  Field_Weakening/3(id_Tgt) -> [id_Tgt]
  [n_motAbs] -> Field_Weakening/2(n_motAbs)
  a_elecAngle/1 -> [a_elecAngle]
  Mux1/1 -> Scope9/1
  Mux2/1 -> Scope9/2
  [Vd_I] -> r_devSignal2/1
  [Vq_I] -> r_devSignal1/1
  [iq] -> FeefForward_Decoupling/2(iq_Tgt)
  [id] -> FeefForward_Decoupling/3(id_Tgt)
  [n_mot] -> FeefForward_Decoupling/1(n_mot)
  FeefForward_Decoupling/2(Vd_Ffwd) -> [Vd_Ffwd]
  FeefForward_Decoupling/1(Vq_Ffwd) -> [Vq_Ffwd]
  [Vd_Ffwd] -> Vd_Calculation/3(Vd_Ffwd)
  [Vq_Ffwd] -> Voltage_Mode/2(Vq_Ffwd)
  [Vq_Ffwd] -> Speed_Mode/2(Vq_Ffwd)
  [Vq_Ffwd] -> Torque_Mode/2(Vq_Ffwd)
  Vd_Calculation/2(Vd_I) -> [Vd_I]
  Torque_Mode/2(Vq_I) -> [Vq_I]
  Field_Weakening/4(id_TgtAbs) -> [id_TgtAbs]
  If2/1 -> FeefForward_Decoupling/Action
  b_FfwdEna/1 -> If2/1
  Torque_Mode/3(iq_Tgt) -> [iq_Tgt]

== system BLDCmotorControl_FOC_R2017b_fixdt_Ffwd/BLDC_controller/BLDC_controller/F05_Control_Type_Management ==
  b_enaFOC : Inport
  z_pos : Inport  Port=2
  z_ctrlTypSel : Inport  Port=3
  r_phaA : Inport  Port=4
  r_phaB : Inport  Port=5
  r_phaC : Inport  Port=6
  Vq : Inport  Port=7
  r_inpTgtSca : Inport  Port=8
  CTRL_COMM1 : Constant  Value=CTRL_COM  OutDataTypeStr=Inherit: Inherit via back propagation
  Demux : Demux  Outputs=3
  Divide2 : Product  Inputs=**  RndMeth=Simplest  OutDataTypeStr=Inherit: Same as first input
  Mux2 : Mux  Inputs=3
  Relational Operator6 : RelationalOperator  Operator=~=  OutDataTypeStr=boolean  RndMeth=Simplest  InputSameDT=off
  Switch1 : Switch  Criteria=u2 ~= 0  OutDataTypeStr=Inherit: Inherit via back propagation  RndMeth=Zero  SaturateOnIntegerOverflow=off  InputSameDT=off
  Switch2 : Switch  Criteria=u2 ~= 0  OutDataTypeStr=Inherit: Inherit via back propagation  RndMeth=Zero  SaturateOnIntegerOverflow=off  InputSameDT=off
  z_commutMap_M1 : LookupNDDirect  InputsSelectThisObjectFromTable=Vector  Table=z_commutMap_M1  DiagnosticForOutOfRangeInput=None  TableDataTypeStr=int16
  DC_phaA : Outport  OutputWhenDisabled=reset  InitialOutput=0  VectorParamsAs1DForOutWhenUnconnected=off
  DC_phaB : Outport  Port=2  OutputWhenDisabled=reset  InitialOutput=0  VectorParamsAs1DForOutWhenUnconnected=off
  "DC_phaC " : Outport  Port=3  OutputWhenDisabled=reset  InitialOutput=0  VectorParamsAs1DForOutWhenUnconnected=off
  wires:
  Demux/3 -> [DC_phaC]
  Demux/2 -> [DC_phaB]
  Demux/1 -> [DC_phaA]
  z_pos/1 -> [z_pos]
  [DC_phaC] -> "DC_phaC "/1
  [DC_phaB] -> DC_phaB/1
  [DC_phaA] -> DC_phaA/1
  [z_pos] -> z_commutMap_M1/1
  Switch1/1 -> Demux/1
  r_phaA/1 -> [r_phaA]
  r_phaB/1 -> [r_phaB]
  r_phaC/1 -> [r_phaC]
  Vq/1 -> [Vq]
  [r_phaA] -> Mux2/1
  [r_phaB] -> Mux2/2
  [r_phaC] -> Mux2/3
  z_commutMap_M1/1 -> Divide2/2
  Divide2/1 -> Switch1/3
  b_enaFOC/1 -> [b_enaFOC]
  Mux2/1 -> Switch1/1
  [b_enaFOC] -> Switch1/2
  Switch2/1 -> Divide2/1
  [Vq] -> Switch2/1
  [z_ctrlTypSel] -> Relational Operator6/1
  CTRL_COMM1/1 -> Relational Operator6/2
  Relational Operator6/1 -> Switch2/2
  r_inpTgtSca/1 -> [r_inpTgtSca]
  [r_inpTgtSca] -> Switch2/3
  z_ctrlTypSel/1 -> [z_ctrlTypSel]

== system BLDCmotorControl_FOC_R2017b_fixdt_Ffwd/BLDC_controller/BLDC_controller/Implemented_control_methods ==

== system BLDCmotorControl_FOC_R2017b_fixdt_Ffwd/PWM_gates/PWM_generator1/__InputSSForSFun__ ==
  DC : Inport  SampleTime=Ts
  __UniqueOutportName__1__ : Outport  VectorParamsAs1DForOutWhenUnconnected=off
  wires:
  DC/1 -> __UniqueOutportName__1__/1

== system BLDCmotorControl_FOC_R2017b_fixdt_Ffwd/PWM_gates/PWM_generator1/__OutputSSForSFun__ ==
  __UniqueInportName__1__ : Inport
  PWM : Outport  VectorParamsAs1DForOutWhenUnconnected=off
  wires:
  __UniqueInportName__1__/1 -> PWM/1

== system BLDCmotorControl_FOC_R2017b_fixdt_Ffwd/PWM_gates/PWM_generator12/__InputSSForSFun__ ==
  DC : Inport  SampleTime=Ts
  __UniqueOutportName__1__ : Outport  VectorParamsAs1DForOutWhenUnconnected=off
  wires:
  DC/1 -> __UniqueOutportName__1__/1

== system BLDCmotorControl_FOC_R2017b_fixdt_Ffwd/PWM_gates/PWM_generator12/__OutputSSForSFun__ ==
  __UniqueInportName__1__ : Inport
  PWM : Outport  VectorParamsAs1DForOutWhenUnconnected=off
  wires:
  __UniqueInportName__1__/1 -> PWM/1

== system BLDCmotorControl_FOC_R2017b_fixdt_Ffwd/PWM_gates/PWM_generator2/__InputSSForSFun__ ==
  DC : Inport  SampleTime=Ts
  __UniqueOutportName__1__ : Outport  VectorParamsAs1DForOutWhenUnconnected=off
  wires:
  DC/1 -> __UniqueOutportName__1__/1

== system BLDCmotorControl_FOC_R2017b_fixdt_Ffwd/PWM_gates/PWM_generator2/__OutputSSForSFun__ ==
  __UniqueInportName__1__ : Inport
  PWM : Outport  VectorParamsAs1DForOutWhenUnconnected=off
  wires:
  __UniqueInportName__1__/1 -> PWM/1

== system BLDCmotorControl_FOC_R2017b_fixdt_Ffwd/PWM_gates/PWM_generator3/__InputSSForSFun__ ==
  DC : Inport  SampleTime=Ts
  __UniqueOutportName__1__ : Outport  VectorParamsAs1DForOutWhenUnconnected=off
  wires:
  DC/1 -> __UniqueOutportName__1__/1

== system BLDCmotorControl_FOC_R2017b_fixdt_Ffwd/PWM_gates/PWM_generator3/__OutputSSForSFun__ ==
  __UniqueInportName__1__ : Inport
  PWM : Outport  VectorParamsAs1DForOutWhenUnconnected=off
  wires:
  __UniqueInportName__1__/1 -> PWM/1

== system BLDCmotorControl_FOC_R2017b_fixdt_Ffwd/PWM_gates/PWM_generator4/__InputSSForSFun__ ==
  DC : Inport  SampleTime=Ts
  __UniqueOutportName__1__ : Outport  VectorParamsAs1DForOutWhenUnconnected=off
  wires:
  DC/1 -> __UniqueOutportName__1__/1

== system BLDCmotorControl_FOC_R2017b_fixdt_Ffwd/PWM_gates/PWM_generator4/__OutputSSForSFun__ ==
  __UniqueInportName__1__ : Inport
  PWM : Outport  VectorParamsAs1DForOutWhenUnconnected=off
  wires:
  __UniqueInportName__1__/1 -> PWM/1

== system BLDCmotorControl_FOC_R2017b_fixdt_Ffwd/PWM_gates/PWM_generator5/__InputSSForSFun__ ==
  DC : Inport  SampleTime=Ts
  __UniqueOutportName__1__ : Outport  VectorParamsAs1DForOutWhenUnconnected=off
  wires:
  DC/1 -> __UniqueOutportName__1__/1

== system BLDCmotorControl_FOC_R2017b_fixdt_Ffwd/PWM_gates/PWM_generator5/__OutputSSForSFun__ ==
  __UniqueInportName__1__ : Inport
  PWM : Outport  VectorParamsAs1DForOutWhenUnconnected=off
  wires:
  __UniqueInportName__1__/1 -> PWM/1

== system BLDCmotorControl_FOC_R2017b_fixdt_Ffwd/BLDC_controller/BLDC_controller/F01_Estimations/F01_01_Edge_Detector ==
  b_hallA : Inport
  b_hallB : Inport  Port=2
  b_hallC : Inport  Port=3
  Bitwise Operator : simulink/Logic and Bit Operations/Bitwise Operator  logicop=XOR  UseBitMask=off  NumInputPorts=6  BitMask=bin2dec('11011001')  BitMaskRealWorld=Stored Integer
  Data Type Conversion2 : DataTypeConversion  OutDataTypeStr=boolean  SaturateOnIntegerOverflow=off  RndMeth=Floor
  UnitDelay1 : UnitDelay  SampleTime=-1  HasFrameUpgradeWarning=on
      settings: AttributesFormatString=Ini=%<X0>
  UnitDelay2 : UnitDelay  SampleTime=-1  HasFrameUpgradeWarning=on
      settings: AttributesFormatString=Ini=%<X0>
  UnitDelay3 : UnitDelay  SampleTime=-1  HasFrameUpgradeWarning=on
      settings: AttributesFormatString=Ini=%<X0>
  "b_edge " : Outport  OutputWhenDisabled=reset  InitialOutput=0  VectorParamsAs1DForOutWhenUnconnected=off
  wires:
  b_hallA/1 -> UnitDelay3/1, Bitwise Operator/1
  b_hallC/1 -> UnitDelay2/1, Bitwise Operator/3
  b_hallB/1 -> UnitDelay1/1, Bitwise Operator/2
  Bitwise Operator/1 -> Data Type Conversion2/1
  UnitDelay1/1 -> Bitwise Operator/5
  UnitDelay2/1 -> Bitwise Operator/6
  UnitDelay3/1 -> Bitwise Operator/4
  Data Type Conversion2/1 -> "b_edge "/1

== system BLDCmotorControl_FOC_R2017b_fixdt_Ffwd/BLDC_controller/BLDC_controller/F01_Estimations/F01_02_Position_Calculation ==
  note: This calculates the low resolution position based on Hall sensors.
  b_hallA : Inport
  b_hallB : Inport  Port=2
  b_hallC : Inport  Port=3
  Selector : Selector  IndexMode=Zero-based  InputPortWidth=length(vec_hallToPos)  IndexOptions=Index vector (port)  Indices=[1 3]  OutputSizes=1
  Sum : Sum  Inputs=+++  RndMeth=Simplest  OutDataTypeStr=Inherit: Same as first input
  g_Ha : Gain  Gain=4  OutDataTypeStr=Inherit: Inherit via back propagation  RndMeth=Zero  ParamDataTypeStr=Inherit: Same as input
  g_Hb : Gain  Gain=2  OutDataTypeStr=Inherit: Inherit via back propagation  RndMeth=Simplest  ParamDataTypeStr=Inherit: Same as input
  vec_hallToPos : Constant  Value=vec_hallToPos  OutDataTypeStr=int8
  z_posRaw : Outport  OutputWhenDisabled=reset  InitialOutput=0  VectorParamsAs1DForOutWhenUnconnected=off
  "z_pos " : Outport  Port=2  OutputWhenDisabled=reset  InitialOutput=0  VectorParamsAs1DForOutWhenUnconnected=off
  wires:
  b_hallC/1 -> Sum/3
  g_Ha/1 -> Sum/1
  g_Hb/1 -> Sum/2
  Sum/1 -> z_posRaw/1, Selector/2
  b_hallA/1 -> g_Ha/1
  b_hallB/1 -> g_Hb/1
  vec_hallToPos/1 -> Selector/1
  Selector/1 -> "z_pos "/1

== system BLDCmotorControl_FOC_R2017b_fixdt_Ffwd/BLDC_controller/BLDC_controller/F01_Estimations/F01_03_Direction_Detection ==
  z_pos : Inport
  Action Port : ActionPort  ActionPortLabel=if(u1 ~= 0)
  Constant20 : Constant  Value=-5  OutDataTypeStr=Inherit: Inherit via back propagation
  Constant23 : Constant  Value=-1  OutDataTypeStr=int8
  Constant24 : Constant  OutDataTypeStr=int8
  Constant8 : Constant  OutDataTypeStr=Inherit: Inherit via back propagation
  Logical Operator3 : Logic  Operator=OR  AllPortsSameDT=off  OutDataTypeStr=boolean
  Relational Operator1 : RelationalOperator  Operator===  OutDataTypeStr=boolean  RndMeth=Simplest  InputSameDT=off
  Relational Operator6 : RelationalOperator  Operator===  OutDataTypeStr=boolean  RndMeth=Simplest  InputSameDT=off
  Sum2 : Sum  Inputs=|+-  InputSameDT=on  RndMeth=Zero  OutDataTypeStr=Inherit: Same as first input
  Switch2 : Switch  Criteria=u2 ~= 0  OutDataTypeStr=Inherit: Inherit via back propagation  RndMeth=Simplest  SaturateOnIntegerOverflow=off  InputSameDT=off
  UnitDelay2 : UnitDelay  SampleTime=-1  HasFrameUpgradeWarning=on
  UnitDelay3 : UnitDelay  SampleTime=-1  HasFrameUpgradeWarning=on
      settings: AttributesFormatString=Ini=%<X0>
  z_dir : Outport  VectorParamsAs1DForOutWhenUnconnected=off
  z_dirPrev : Outport  Port=2  VectorParamsAs1DForOutWhenUnconnected=off
  wires:
  UnitDelay2/1 -> Sum2/2
  Relational Operator1/1 -> Logical Operator3/1
  Constant8/1 -> Relational Operator1/2
  Sum2/1 -> Relational Operator6/1, Relational Operator1/1
  Relational Operator6/1 -> Logical Operator3/2
  Constant20/1 -> Relational Operator6/2
  Constant24/1 -> Switch2/1
  Constant23/1 -> Switch2/3
  Logical Operator3/1 -> Switch2/2
  z_pos/1 -> Sum2/1, UnitDelay2/1
  Switch2/1 -> UnitDelay3/1, z_dir/1
  UnitDelay3/1 -> z_dirPrev/1

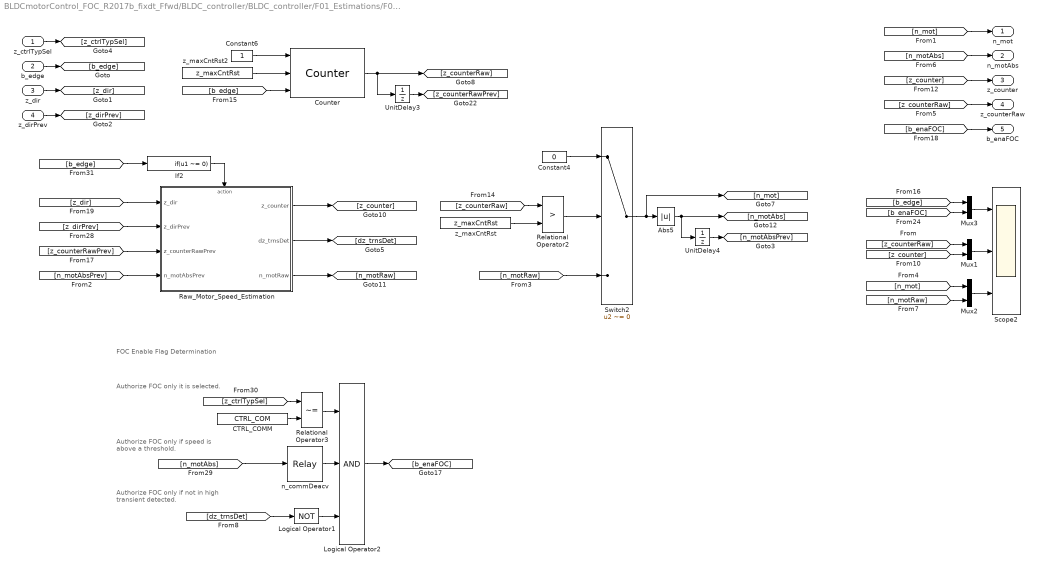
== system BLDCmotorControl_FOC_R2017b_fixdt_Ffwd/BLDC_controller/BLDC_controller/F01_Estimations/F01_04_Speed_Estimation ==
  note: FOC Enable Flag Determination
  note: Authorize FOC only if speed is above a threshold.
  note: Authorize FOC only if not in high transient detected.
  note: Authorize FOC only it is selected.
  z_ctrlTypSel : Inport
  b_edge : Inport  Port=2
  z_dir : Inport  Port=3
  z_dirPrev : Inport  Port=4
  Abs5 : Abs  OutDataTypeStr=Inherit: Inherit via back propagation  RndMeth=Zero  SaturateOnIntegerOverflow=off
  CTRL_COMM : Constant  Value=CTRL_COM  OutDataTypeStr=Inherit: Inherit via back propagation
  Constant4 : Constant  Value=0  OutDataTypeStr=Inherit: Inherit via back propagation
  Constant6 : Constant  OutDataTypeStr=fixdt(1,16,0)
  Counter : BLDC_controller_Lib/Counter  z_cntInit=z_maxCntRst
      settings: AttributesFormatString=Ini=%<z_cntInit>
  If2 : If  IfExpression=u1 ~= 0  ShowElse=off
  Logical Operator1 : Logic  Operator=NOT  AllPortsSameDT=off  OutDataTypeStr=boolean
  Logical Operator2 : Logic  Inputs=3  AllPortsSameDT=off  OutDataTypeStr=boolean
  Mux1 : Mux  Inputs=2
  Mux2 : Mux  Inputs=2
  Mux3 : Mux  Inputs=2
  Raw_Motor_Speed_Estimation : Subsystem
  Relational Operator2 : RelationalOperator  Operator=>  OutDataTypeStr=boolean  RndMeth=Simplest  InputSameDT=off
  Relational Operator3 : RelationalOperator  Operator=~=  OutDataTypeStr=boolean  RndMeth=Simplest  InputSameDT=off
  Scope2 : Scope  NumInputPorts=3
      settings: ActiveDisplayYMinimum=-0.125  ActiveDisplayYMaximum=1.125
  Switch2 : Switch  Criteria=u2 ~= 0  OutDataTypeStr=Inherit: Inherit via back propagation  RndMeth=Zero  SaturateOnIntegerOverflow=off  InputSameDT=off
  UnitDelay3 : UnitDelay  InitialCondition=z_maxCntRst  SampleTime=-1  HasFrameUpgradeWarning=on
      settings: AttributesFormatString=Ini=%<X0>
  UnitDelay4 : UnitDelay  SampleTime=-1  HasFrameUpgradeWarning=on
      settings: AttributesFormatString=Ini=%<X0>
  n_commDeacv : Relay  OnSwitchValue=n_commDeacvHi  OffSwitchValue=n_commAcvLo  OutDataTypeStr=boolean
  z_maxCntRst : Constant  Value=z_maxCntRst  OutDataTypeStr=Inherit: Inherit via back propagation
  z_maxCntRst2 : Constant  Value=z_maxCntRst  OutDataTypeStr=Inherit: Inherit via back propagation
  n_mot : Outport  VectorParamsAs1DForOutWhenUnconnected=off
  n_motAbs : Outport  Port=2  VectorParamsAs1DForOutWhenUnconnected=off
  z_counter : Outport  Port=3  OutputWhenDisabled=reset  InitialOutput=0  VectorParamsAs1DForOutWhenUnconnected=off
  z_counterRaw : Outport  Port=4  OutputWhenDisabled=reset  InitialOutput=0  VectorParamsAs1DForOutWhenUnconnected=off
  b_enaFOC : Outport  Port=5  VectorParamsAs1DForOutWhenUnconnected=off
  wires:
  [n_motRaw] -> Mux2/2
  Mux2/1 -> Scope2/3
  [n_mot] -> Mux2/1
  Mux1/1 -> Scope2/2
  [z_counterRaw] -> Mux1/1
  [z_counter] -> Mux1/2
  b_edge/1 -> [b_edge]
  [n_mot] -> n_mot/1
  z_dir/1 -> [z_dir]
  [z_counter] -> z_counter/1
  [z_counterRaw] -> z_counterRaw/1
  UnitDelay3/1 -> [z_counterRawPrev]
  z_dirPrev/1 -> [z_dirPrev]
  [z_dir] -> Raw_Motor_Speed_Estimation/1(z_dir)
  Abs5/1 -> UnitDelay4/1, [n_motAbs]
  Raw_Motor_Speed_Estimation/1(z_counter) -> [z_counter]
  [z_dirPrev] -> Raw_Motor_Speed_Estimation/2(z_dirPrev)
  If2/1 -> Raw_Motor_Speed_Estimation/Action
  [z_counterRawPrev] -> Raw_Motor_Speed_Estimation/3(z_counterRawPrev)
  [b_enaFOC] -> b_enaFOC/1
  z_ctrlTypSel/1 -> [z_ctrlTypSel]
  [z_counterRaw] -> Relational Operator2/1
  z_maxCntRst/1 -> Relational Operator2/2
  Constant4/1 -> Switch2/1
  Raw_Motor_Speed_Estimation/3(n_motRaw) -> [n_motRaw]
  Switch2/1 -> [n_mot], Abs5/1
  Mux3/1 -> Scope2/1
  [b_enaFOC] -> Mux3/2
  [b_edge] -> Mux3/1
  [b_edge] -> If2/1
  Relational Operator2/1 -> Switch2/2
  UnitDelay4/1 -> [n_motAbsPrev]
  [n_motAbsPrev] -> Raw_Motor_Speed_Estimation/4(n_motAbsPrev)
  [n_motAbs] -> n_motAbs/1
  CTRL_COMM/1 -> Relational Operator3/2
  [z_ctrlTypSel] -> Relational Operator3/1
  [n_motAbs] -> n_commDeacv/1
  Raw_Motor_Speed_Estimation/2(dz_trnsDet) -> [dz_trnsDet]
  Relational Operator3/1 -> Logical Operator2/1
  n_commDeacv/1 -> Logical Operator2/2
  Logical Operator1/1 -> Logical Operator2/3
  Logical Operator2/1 -> [b_enaFOC]
  [dz_trnsDet] -> Logical Operator1/1
  [n_motRaw] -> Switch2/3
  z_maxCntRst2/1 -> Counter/2
  [b_edge] -> Counter/3
  Constant6/1 -> Counter/1
  Counter/1 -> UnitDelay3/1, [z_counterRaw]

== system BLDCmotorControl_FOC_R2017b_fixdt_Ffwd/BLDC_controller/BLDC_controller/F01_Estimations/F01_05_Electrical_Angle_Estimation ==
  note: Electrical angle calculation
  note: This switch is to manage the situation when FOC control method is not enabled.
  z_pos : Inport
  z_dir : Inport  Port=2
  z_counter : Inport  Port=3
  z_counterRaw : Inport  Port=4
  b_enaFOC : Inport  Port=5
  Constant16 : Constant  OutDataTypeStr=Inherit: Inherit via back propagation
  Constant2 : Constant  OutDataTypeStr=Inherit: Inherit via back propagation
  Divide4 : Product  Inputs=*/*  RndMeth=Simplest  SaturateOnIntegerOverflow=on  OutDataTypeStr=Inherit: Same as first input
  Divide5 : Product  Inputs=**  RndMeth=Simplest  OutDataTypeStr=Inherit: Same as first input
  Mux : Mux  Inputs=3
  Product6 : Product  OutDataTypeStr=Inherit: Inherit via back propagation  RndMeth=Simplest
  Relational Operator7 : RelationalOperator  Operator===  OutDataTypeStr=boolean  RndMeth=Simplest  InputSameDT=off
  Scope : Scope  NumInputPorts=2
      settings: ActiveDisplayYMinimum=-45.52734  ActiveDisplayYMaximum=409.74609
  Sum1 : Sum  RndMeth=Simplest  OutDataTypeStr=Inherit: Same as first input
  Sum2 : Sum  RndMeth=Simplest  OutDataTypeStr=Inherit: Same as first input
  Switch1 : Switch  Criteria=u2 ~= 0  OutDataTypeStr=Inherit: Inherit via back propagation  RndMeth=Zero  SaturateOnIntegerOverflow=off  InputSameDT=off
  Switch3 : Switch  Criteria=u2 ~= 0  OutDataTypeStr=Inherit: Inherit via back propagation  RndMeth=Zero  SaturateOnIntegerOverflow=off  InputSameDT=off
  a_elecAngle1 : Constant  Value=a_elecAngle  OutDataTypeStr=fixdt(1,16,6)
  a_elecAngle : Outport  OutputWhenDisabled=reset  InitialOutput=0  VectorParamsAs1DForOutWhenUnconnected=off
  wires:
  z_pos/1 -> [z_pos]
  z_dir/1 -> [z_dir]
  Mux/1 -> Scope/1
  [b_enaFOC] -> Scope/2
  z_counterRaw/1 -> [z_counterRaw]
  z_counter/1 -> [z_counter]
  [z_counter] -> Divide4/2
  Switch3/1 -> Divide5/2
  [z_pos] -> Switch3/1, Sum1/1
  Constant2/1 -> Sum1/2
  Product6/1 -> Sum2/2
  Relational Operator7/1 -> Switch3/2
  Constant16/1 -> Relational Operator7/2
  a_elecAngle1/1 -> Divide5/1, Divide4/1
  [z_dir] -> Relational Operator7/1
  Sum1/1 -> Switch3/3
  Divide4/1 -> Product6/1
  Divide5/1 -> [a_elecAngleLowRes], Sum2/1
  b_enaFOC/1 -> [b_enaFOC]
  [b_enaFOC] -> Switch1/2
  Sum2/1 -> [a_elecAngleRaw]
  [a_elecAngleRaw] -> Switch1/1
  [a_elecAngleLowRes] -> Switch1/3
  [z_dir] -> Product6/2
  [z_counterRaw] -> Divide4/3
  [a_elecAngle] -> a_elecAngle/1
  Switch1/1 -> [a_elecAngle]
  [a_elecAngle] -> Mux/3
  [a_elecAngleLowRes] -> Mux/2
  [a_elecAngleRaw] -> Mux/1

== system BLDCmotorControl_FOC_R2017b_fixdt_Ffwd/BLDC_controller/BLDC_controller/F03_Control_Mode_Manager/Commutation_Control_Type ==
  r_inpTgt : Inport
  Action Port : ActionPort  InitializeStates=reset  ActionPortLabel=if { }
  r_inpTgtScaCOM : Outport  VectorParamsAs1DForOutWhenUnconnected=off
  wires:
  r_inpTgt/1 -> r_inpTgtScaCOM/1

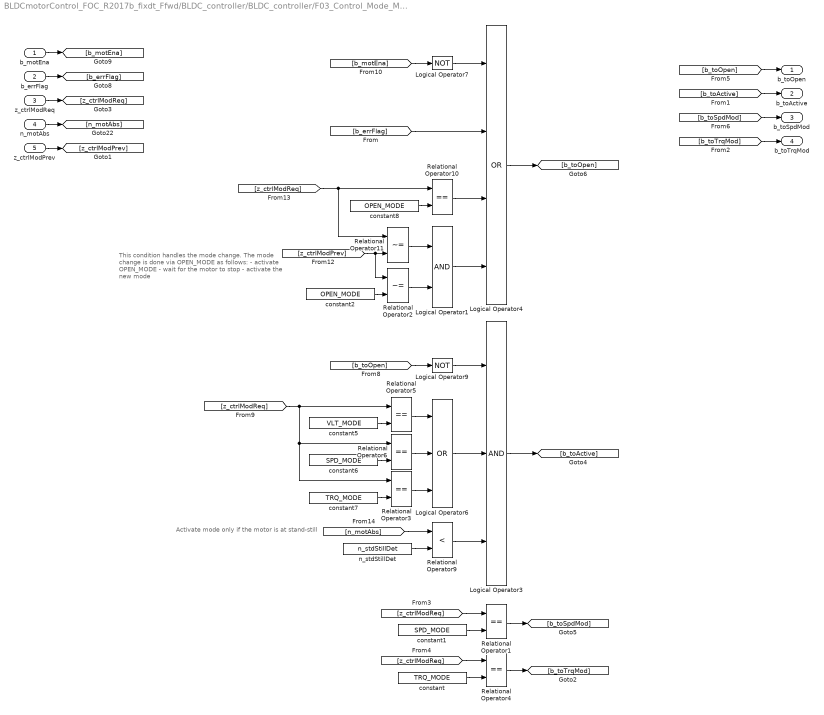
== system BLDCmotorControl_FOC_R2017b_fixdt_Ffwd/BLDC_controller/BLDC_controller/F03_Control_Mode_Manager/F02_01_Mode_Transition_Calculation ==
  note: This condition handles the mode change. The mode change is done via OPEN_MODE as follows:
      | - activate OPEN_MODE
      | - wait for the motor to stop
      | - activate the new mode
  note: Activate mode only if the motor is at stand-still
  b_motEna : Inport
  b_errFlag : Inport  Port=2
  z_ctrlModReq : Inport  Port=3
  n_motAbs : Inport  Port=4
  z_ctrlModPrev : Inport  Port=5
  Logical Operator1 : Logic  AllPortsSameDT=off  OutDataTypeStr=boolean
  Logical Operator3 : Logic  Inputs=3  AllPortsSameDT=off  OutDataTypeStr=boolean
  Logical Operator4 : Logic  Operator=OR  Inputs=4  AllPortsSameDT=off  OutDataTypeStr=boolean
  Logical Operator6 : Logic  Operator=OR  Inputs=3  AllPortsSameDT=off  OutDataTypeStr=boolean
  Logical Operator7 : Logic  Operator=NOT  AllPortsSameDT=off  OutDataTypeStr=boolean
  Logical Operator9 : Logic  Operator=NOT  AllPortsSameDT=off  OutDataTypeStr=boolean
  Relational Operator{1,3..6,10} (6 alike) : RelationalOperator  Operator===  OutDataTypeStr=boolean  RndMeth=Simplest  InputSameDT=off
  Relational Operator11 : RelationalOperator  Operator=~=  OutDataTypeStr=boolean  RndMeth=Simplest  InputSameDT=off
  Relational Operator2 : RelationalOperator  Operator=~=  OutDataTypeStr=boolean  RndMeth=Simplest  InputSameDT=off
  Relational Operator9 : RelationalOperator  Operator=<  OutDataTypeStr=boolean  RndMeth=Simplest  InputSameDT=off
  constant : Constant  Value=TRQ_MODE  OutDataTypeStr=Inherit: Inherit via back propagation
  constant1 : Constant  Value=SPD_MODE  OutDataTypeStr=Inherit: Inherit via back propagation
  constant2 : Constant  Value=OPEN_MODE  OutDataTypeStr=Inherit: Inherit via back propagation
  constant5 : Constant  Value=VLT_MODE  OutDataTypeStr=Inherit: Inherit via back propagation
  constant6 : Constant  Value=SPD_MODE  OutDataTypeStr=Inherit: Inherit via back propagation
  constant7 : Constant  Value=TRQ_MODE  OutDataTypeStr=Inherit: Inherit via back propagation
  constant8 : Constant  Value=OPEN_MODE  OutDataTypeStr=Inherit: Inherit via back propagation
  n_stdStillDet : Constant  Value=n_stdStillDet  OutDataTypeStr=Inherit: Inherit via back propagation
  b_toOpen : Outport  OutputWhenDisabled=reset  InitialOutput=0  VectorParamsAs1DForOutWhenUnconnected=off
  b_toActive : Outport  Port=2  OutputWhenDisabled=reset  InitialOutput=0  VectorParamsAs1DForOutWhenUnconnected=off
  b_toSpdMod : Outport  Port=3  OutputWhenDisabled=reset  InitialOutput=0  VectorParamsAs1DForOutWhenUnconnected=off
  b_toTrqMod : Outport  Port=4  OutputWhenDisabled=reset  InitialOutput=0  VectorParamsAs1DForOutWhenUnconnected=off
  wires:
  Relational Operator6/1 -> Logical Operator6/2
  constant6/1 -> Relational Operator6/2
  constant7/1 -> Relational Operator3/2
  Relational Operator3/1 -> Logical Operator6/3
  Relational Operator4/1 -> [b_toTrqMod]
  Logical Operator3/1 -> [b_toActive]
  [n_motAbs] -> Relational Operator9/1
  [z_ctrlModReq] -> Relational Operator11/1, Relational Operator10/1
  constant5/1 -> Relational Operator5/2
  [z_ctrlModReq] -> Relational Operator4/1
  constant/1 -> Relational Operator4/2
  constant1/1 -> Relational Operator1/2
  Relational Operator1/1 -> [b_toSpdMod]
  n_stdStillDet/1 -> Relational Operator9/2
  [z_ctrlModReq] -> Relational Operator1/1
  Relational Operator5/1 -> Logical Operator6/1
  [z_ctrlModReq] -> Relational Operator6/1, Relational Operator3/1, Relational Operator5/1
  Logical Operator9/1 -> Logical Operator3/1
  constant2/1 -> Relational Operator2/2
  Relational Operator10/1 -> Logical Operator4/3
  [z_ctrlModPrev] -> Relational Operator2/1, Relational Operator11/2
  [b_motEna] -> Logical Operator7/1
  [b_toOpen] -> Logical Operator9/1
  Logical Operator4/1 -> [b_toOpen]
  Relational Operator2/1 -> Logical Operator1/2
  Relational Operator11/1 -> Logical Operator1/1
  Logical Operator6/1 -> Logical Operator3/2
  constant8/1 -> Relational Operator10/2
  Logical Operator1/1 -> Logical Operator4/4
  Logical Operator7/1 -> Logical Operator4/1
  Relational Operator9/1 -> Logical Operator3/3
  n_motAbs/1 -> [n_motAbs]
  b_motEna/1 -> [b_motEna]
  z_ctrlModReq/1 -> [z_ctrlModReq]
  z_ctrlModPrev/1 -> [z_ctrlModPrev]
  [b_toOpen] -> b_toOpen/1
  [b_toActive] -> b_toActive/1
  [b_toTrqMod] -> b_toTrqMod/1
  [b_toSpdMod] -> b_toSpdMod/1
  b_errFlag/1 -> [b_errFlag]
  [b_errFlag] -> Logical Operator4/2

== system BLDCmotorControl_FOC_R2017b_fixdt_Ffwd/BLDC_controller/BLDC_controller/F03_Control_Mode_Manager/FOC_Control_Type ==
  r_inpTgt : Inport
  z_ctrlMod : Inport  Port=2
  Action Port : ActionPort  InitializeStates=reset  ActionPortLabel=else { }
  Divide1 : Product  Inputs=**  OutDataTypeStr=fixdt(1,16,4)  RndMeth=Simplest
  Divide4 : Product  Inputs=*/  OutDataTypeStr=fixdt(0,16,12)  RndMeth=Simplest
  Mux : Mux
  Selector : Selector  IndexMode=Zero-based  InputPortWidth=4  IndexOptions=Index vector (port)  Indices=[1 3]  OutputSizes=1
  Vd_max : Constant  Value=Vd_max  OutDataTypeStr=fixdt(1,16,4)
  constant : Constant  Value=1000  OutDataTypeStr=Inherit: Inherit via back propagation
  constant1 : Constant  Value=0  OutDataTypeStr=Inherit: Inherit via back propagation
  i_max : Constant  Value=i_max  OutDataTypeStr=fixdt(1,16,4)
  n_max : Constant  Value=n_max  OutDataTypeStr=fixdt(1,16,4)
  r_inpTgtScaFOC : Outport  VectorParamsAs1DForOutWhenUnconnected=off
  wires:
  r_inpTgt/1 -> [r_inpTgt]
  [r_inpTgtScaFOC] -> r_inpTgtScaFOC/1
  z_ctrlMod/1 -> [z_ctrlMod]
  constant/1 -> Divide4/2
  Selector/1 -> Divide4/1
  constant1/1 -> Mux/1
  i_max/1 -> Mux/4
  Vd_max/1 -> Mux/2
  Mux/1 -> Selector/1
  n_max/1 -> Mux/3
  [z_ctrlMod] -> Selector/2
  Divide4/1 -> Divide1/2
  Divide1/1 -> [r_inpTgtScaFOC]
  [r_inpTgt] -> Divide1/1
